simulink model "resonant_PI_ctrl_2022_03_08"  (R2021b)
settings: Solver=VariableStepAuto  StartTime=0.0  StopTime=simlegth  RelTol=1e-3
values from neighbouring files (symbols this model uses):
  Ad = [cos(w*ts) sin(w*ts)/w; -w*sin(w*ts) cos(w*ts)]    [pres_ctrl_design.m]    (also in resonant_PI.m = [cos(w*Ts) sin(w*Ts)/w; -w*sin(w*Ts) cos(w*Ts)])
  Bd = [(1-cos(w*ts))/w^2 sin(w*ts)/w]'    [pres_ctrl_design.m]    (also in resonant_PI.m = [(1-cos(w*Ts))/w^2 sin(w*Ts)/w]')
  C = [0 1]    [pres_ctrl_design.m]    (also in resonant_PI.m)
  ki = 18    [pres_ctrl_design.m]    (also in resonant_PI.m = 8)
  kp = 0.5    [pres_ctrl_design.m]    (also in resonant_PI.m = 0.1)
  Tc = ts/10    (= 0.0001)    [pres_ctrl_design.m]    (also in resonant_PI.m = 1e-05)
  ts = 1e-3    (= 0.001)    [pres_ctrl_design.m]
  w = 2*pi*50    (= 314.159265359)    [pres_ctrl_design.m]    (also in resonant_PI.m)
libraries: cstblocks x2
settings Model: Creator=dabagnara  LastModifiedBy=dabagnara
settings SolverCC: AlgebraicLoopSolver=TrustRegion
settings DataIOCC: ReturnWorkspaceOutputs=off
settings DebuggingCC: SFMachineParentedDataDiag=warning

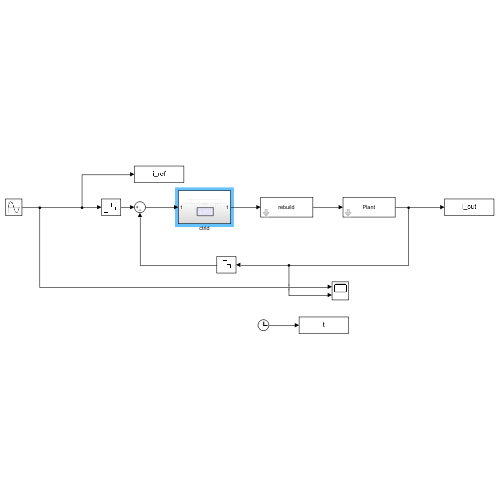
[thumbnail: Simulink's stored preview of the top-level diagram]
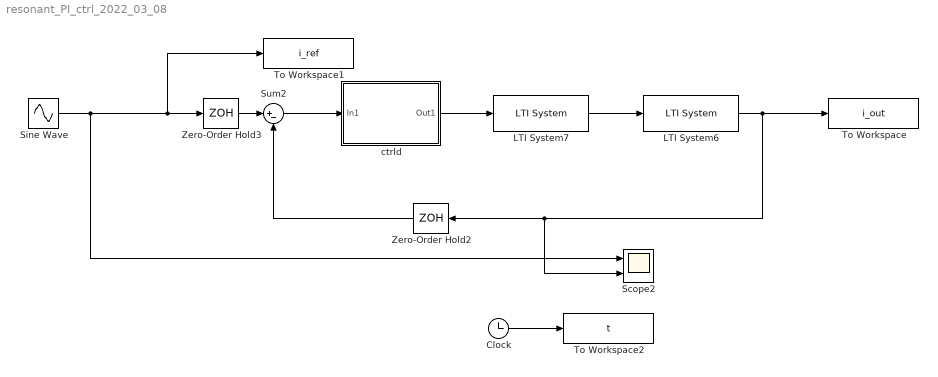
== system resonant_PI_ctrl_2022_03_08 ==
  Clock : Clock
  LTI System6 : cstblocks/LTI System  sys=Plant  IC=[]
  LTI System7 : cstblocks/LTI System  sys=rebuild  IC=[0]
  Scope2 : Scope  NumInputPorts=2
  Sine Wave : Sin  Frequency=w  SampleTime=0
  Sum2 : Sum  Inputs=|+-
  To Workspace : ToWorkspace  VariableName=i_out  SampleTime=Tc
  To Workspace1 : ToWorkspace  VariableName=i_ref  SampleTime=Tc
  To Workspace2 : ToWorkspace  VariableName=t  SampleTime=Tc
  Zero-Order Hold2 : ZeroOrderHold  SampleTime=ts
  Zero-Order Hold3 : ZeroOrderHold  SampleTime=ts
  ctrld : Subsystem
  wires:
  LTI System7/1 -> LTI System6/1
  Zero-Order Hold3/1 -> Sum2/1
  Zero-Order Hold2/1 -> Sum2/2
  Sine Wave/1 -> To Workspace1/1, Zero-Order Hold3/1, Scope2/1
  LTI System6/1 -> Scope2/2, Zero-Order Hold2/1, To Workspace/1
  Sum2/1 -> ctrld/1(In1)
  ctrld/1(Out1) -> LTI System7/1
  Clock/1 -> To Workspace2/1

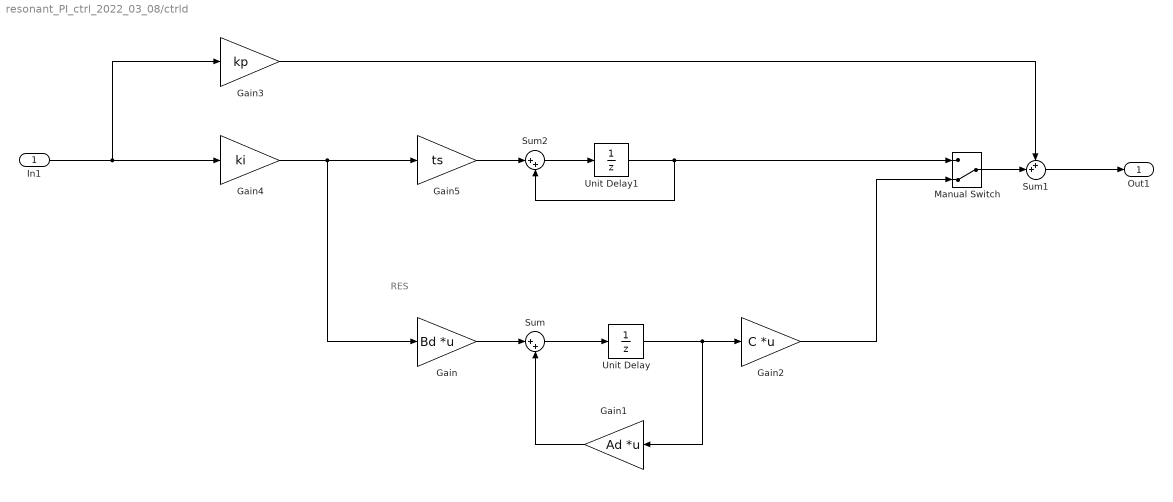
== system resonant_PI_ctrl_2022_03_08/ctrld ==
  note: RES
  In1 : Inport
  Gain : Gain  Gain=Bd  Multiplication=Matrix(K*u)
  Gain1 : Gain  Gain=Ad  Multiplication=Matrix(K*u)
  Gain2 : Gain  Gain=C  Multiplication=Matrix(K*u)
  Gain3 : Gain  Gain=kp
  Gain4 : Gain  Gain=ki
  Gain5 : Gain  Gain=ts
  Manual Switch : ManualSwitch  CurrentSetting=0
  Sum : Sum  Inputs=|++
  Sum1 : Sum  Inputs=++|
  Sum2 : Sum  Inputs=|++
  Unit Delay : UnitDelay  SampleTime=ts  HasFrameUpgradeWarning=on
  Unit Delay1 : UnitDelay  SampleTime=ts  HasFrameUpgradeWarning=on
  Out1 : Outport
  wires:
  In1/1 -> Gain4/1, Gain3/1
  Sum/1 -> Unit Delay/1
  Gain/1 -> Sum/1
  Gain1/1 -> Sum/2
  Unit Delay/1 -> Gain2/1, Gain1/1
  Gain4/1 -> Gain5/1, Gain/1
  Sum1/1 -> Out1/1
  Gain3/1 -> Sum1/1
  Manual Switch/1 -> Sum1/2
  Gain2/1 -> Manual Switch/2
  Unit Delay1/1 -> Sum2/2, Manual Switch/1
  Sum2/1 -> Unit Delay1/1
  Gain5/1 -> Sum2/1
